simulink model "DPT_model"  (R2021b)
settings: Solver=VariableStepAuto  StartTime=0.0  StopTime=0.2  RelTol=1e-3
values from neighbouring files (symbols this model uses):
  Jn = 2*Jd    (= 0.000334)    [lab_4_tf_dpt.m]
  ke = (Un-R*In)/wn    (= 0.320333333333)    [lab_4_tf_dpt.m]
  km = Mn/In    (= 0.228971962617)    [lab_4_tf_dpt.m]
  ku = 20    [lab_4_tf_dpt.m]
  L = 10^-3 * 58    (= 0.058)    [lab_4_tf_dpt.m]
  R = 8.5    [lab_4_tf_dpt.m]
settings Model: Creator=vkad  LastModifiedBy=79159

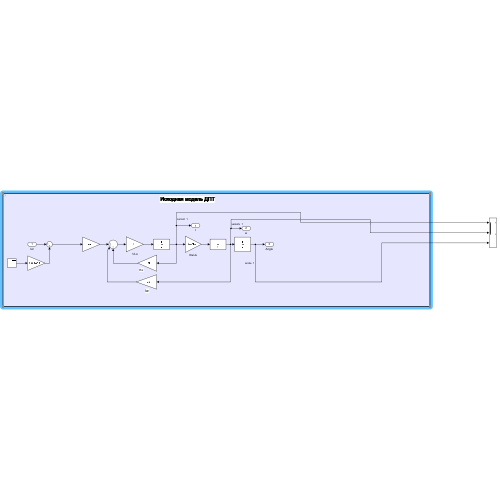
[thumbnail: Simulink's stored preview of the top-level diagram]
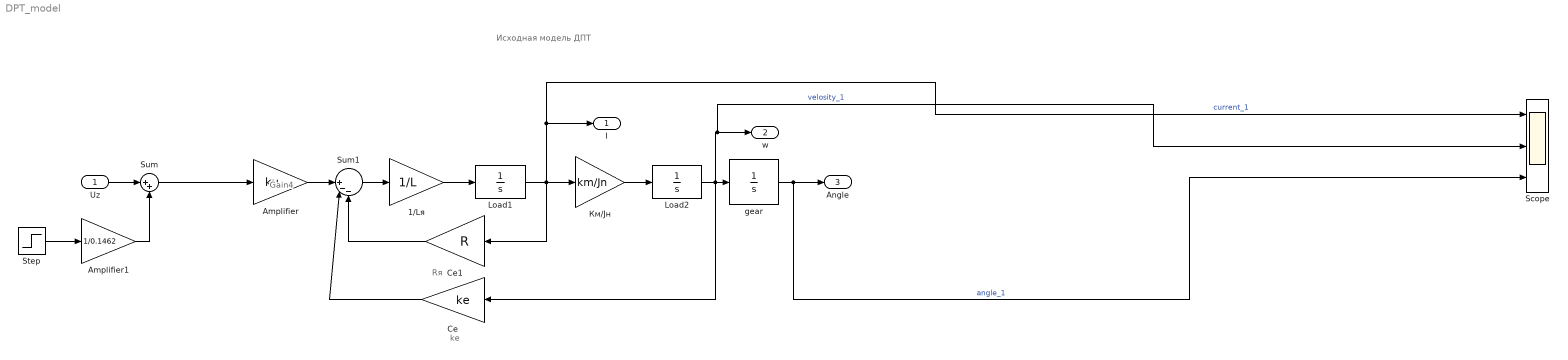
== system DPT_model ==
  note: Rя
  note: Исходная модель ДПТ
  note: Gain4
  note: kе
  Uz : Inport
  1/Lя : Gain  Gain=1/L
  Amplifier : Gain  Gain=ku
  Amplifier1 : Gain  Gain=1/0.1462
  Ce : Gain  Gain=ke
  Ce1 : Gain  Gain=R
  Load1 : TransferFcn  Denominator=[1 0]
  Load2 : TransferFcn  Denominator=[1 0]
  Scope : Scope  NumInputPorts=3
  Step : Step  Time=0  SampleTime=0
  Sum : Sum  Inputs=|++
  Sum1 : Sum  Inputs=||+--
  gear : TransferFcn  Numerator=1  Denominator=[1 0]
  Км/Jн : Gain  Gain=km/Jn
  I : Outport
  w : Outport  Port=2
  Angle : Outport  Port=3
  wires:
  Км/Jн/1 -> Load2/1
  Ce/1 -> Sum1/2
  1/Lя/1 -> Load1/1
  Uz/1 -> Sum/1
  Ce1/1 -> Sum1/3
  gear/1 -> Scope/3, Angle/1  "angle_1"
  Step/1 -> Amplifier1/1
  Amplifier/1 -> Sum1/1
  Sum1/1 -> 1/Lя/1
  Load2/1 -> Scope/2, w/1, Ce/1, gear/1  "velosity_1"
  Load1/1 -> Ce1/1, Км/Jн/1, Scope/1, I/1  "current_1"
  Amplifier1/1 -> Sum/2
  Sum/1 -> Amplifier/1
